simulink library "senseo_lib"  (R2018a)
settings: Solver=VariableStepAuto  StartTime=0.0  StopTime=10.0  RelTol=1e-3
libraries: fl_lib x10, elec_lib x8, $bdroot x2
settings Model: Creator=ChLan  LastModifiedBy=ChLan

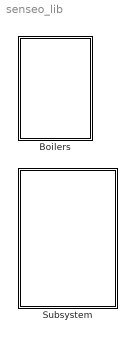
== system senseo_lib ==
  Boilers : Subsystem
  Subsystem : Subsystem

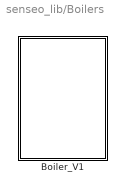
== system senseo_lib/Boilers ==
  Boiler_V1 : Subsystem

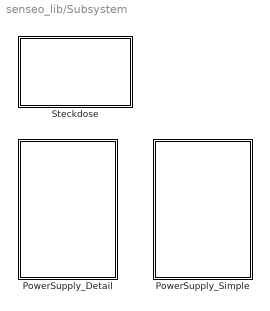
== system senseo_lib/Subsystem ==
  PowerSupply_Detail : Subsystem
  PowerSupply_Simple : Subsystem  VariantControl=1==1
  Steckdose : Subsystem

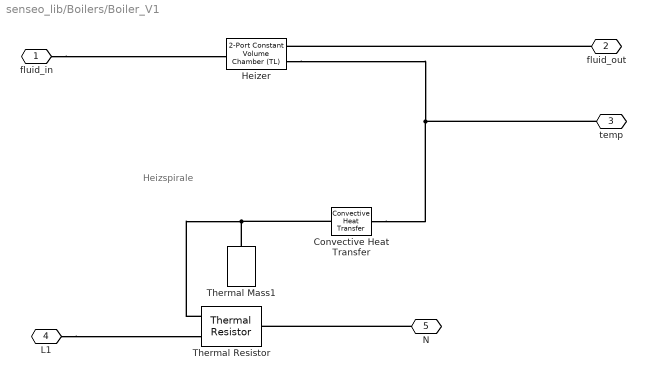
== system senseo_lib/Boilers/Boiler_V1 ==
  note: Heizspirale
  Convective Heat Transfer : fl_lib/Thermal/Thermal Elements/Convective Heat Transfer  area=1000 cm^2  heat_tr_coeff=1000 W/(m^2 * K)  T_specify=off  T_priority=None  T=0 K  T_nominal_specify=off  T_nominal_unit=K  T_nominal_value=1  Q_specify=off  Q_priority=None  Q=0 W  Q_nominal_specify=off  Q_nominal_unit=W  Q_nominal_value=1
  Heizer : fl_lib/Thermal Liquid/Elements/2-Port Constant Volume Chamber (TL)  volume=0.25 l  area_A=0.01 m^2  area_B=0.01 m^2  p_chamber_specify=off  p_chamber_priority=High  p_chamber=0.101325 MPa  p_chamber_nominal_specify=off  p_chamber_nominal_unit=MPa  p_chamber_nominal_value=1  T_chamber_specify=on  T_chamber_priority=High  T_chamber=300 K  T_chamber_nominal_specify=off  T_chamber_nominal_unit=K  T_chamber_nominal_value=1  u_chamber_specify=off  u_chamber_priority=None  u_chamber=83.90600000000001 kJ/kg  u_chamber_nominal_specify=off  u_chamber_nominal_unit=kJ/kg  u_chamber_nominal_value=1  rho_specify=off  rho_priority=None  rho=998.21 kg/m^3  rho_nominal_specify=off  rho_nominal_unit=kg/m^3  rho_nominal_value=1
      settings: SourceProductName=Simscape  SourceProductBaseCode=SS
  Thermal Mass1 : fl_lib/Thermal/Thermal Elements/Thermal Mass  mass=0.05 kg  sp_heat=447 J/kg/K  T_specify=off  T_priority=High  T=300 K  T_nominal_specify=off  T_nominal_unit=K  T_nominal_value=1  Q_specify=off  Q_priority=None  Q=0 W  Q_nominal_specify=off  Q_nominal_unit=W  Q_nominal_value=1
  Thermal Resistor : fl_lib/Electrical/Electrical Elements/Thermal Resistor  R0=35 Ohm  T0=298.15 K  alpha=50e-6 1/K  tc=10 s  K_d=1e-3 W/K  T_specify=off  T_priority=High  T=300 K  T_nominal_specify=off  T_nominal_unit=K  T_nominal_value=1
      settings: SourceProductName=Simscape  SourceProductBaseCode=SS
  fluid_in : PMIOPort  Side=Left
  fluid_out : PMIOPort  Port=2  Side=Right
  temp : PMIOPort  Port=3  Side=Right
  L1 : PMIOPort  Port=4  Side=Left
  N : PMIOPort  Port=5  Side=Right
  connections:
  fluid_in/RConn1 -- Heizer/RConn1
  fluid_out/RConn1 -- Heizer/LConn1
  N/RConn1 -- Thermal Resistor/RConn1
  Convective Heat Transfer/LConn1 -- Thermal Mass1/LConn1 -- Thermal Resistor/LConn1
  temp/RConn1 -- Heizer/LConn2 -- Convective Heat Transfer/RConn1
  L1/RConn1 -- Thermal Resistor/LConn2

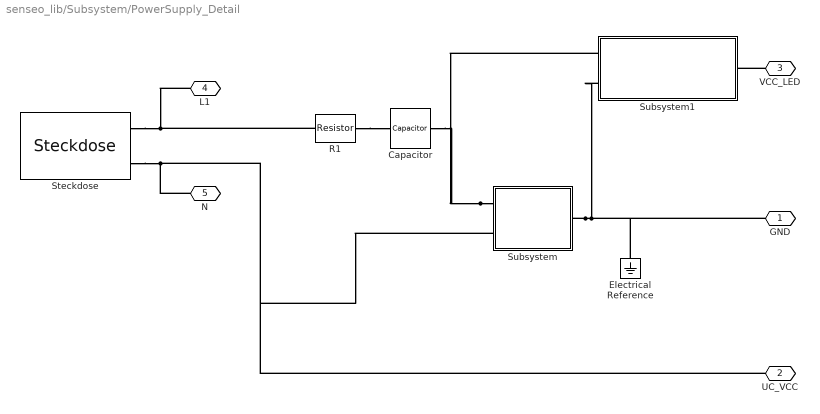
== system senseo_lib/Subsystem/PowerSupply_Detail ==
  Capacitor : elec_lib/Passive Devices/Capacitor  enable_table=0  c=680 nF  Cvec=[1e-05, 1e-06] F  Vvec=[0, 10] V  CV_table_symmetry=1  C_tol=5  enable_C_tol=0  tol_distribution=1  nSigma=4  r=1e-6 Ohm  g=0 1/Ohm  enable_operating_limits=0  operating_limit_action=2  max_working_voltage_range=[-25, 25] V  power_rating=1 W  enable_faults=0  fault_action=1  Cscale_faulted=100  R_faulted=1e-3 Ohm  G_faulted=0 1/Ohm  tau_fault=1e-3 s  enable_temporal_fault=0  t_fault=1 s  enable_behavioral_fault=0  max_permissible_voltage_range=[-100, 100] V  t_fail_on_voltage=1 s  i_specify=off  i_priority=None  i=0 A  i_nominal_specify=off  i_nominal_unit=A  i_nominal_value=1  v_specify=off  v_priority=None  v=0 V  v_nominal_specify=off  v_nominal_unit=V  v_nominal_value=1  vc_specify=off  vc_priority=High  vc=0 V  vc_nominal_specify=off  vc_nominal_unit=V  vc_nominal_value=1
      settings: AttributesFormatString=%<c> %<c_unit>
  Electrical Reference : fl_lib/Electrical/Electrical Elements/Electrical Reference
  R1 : elec_lib/Passive Devices/Resistor  R=100 Ohm  R_tol=5  enable_R_tol=0  tol_distribution=1  nSigma=4  enable_operating_limits=0  operating_limit_action=2  max_working_voltage=100 V  power_rating=1 W  enable_faults=0  fault_action=1  R_faulted=inf Ohm  enable_temporal_fault=0  t_fault=1 s  enable_behavioral_fault=0  max_permissible_current=1 A  t_fail_on_current=1 s  noise_mode=0  sample_time=1e-3 s  repeatability=1  auto_seed=1399327243  user_seed=0  Tdevice=25 degC  alpha=3.93e-3 1/K  Tmeas=25 degC  thermal_mass=100 J/K  power_derating_T1=70 degC  power_derating_T2=155 degC  operating_temperature_range_vec=[-50, 150] degC  temperature_specify=off  temperature_priority=High  temperature=298.15 K  temperature_nominal_specify=off  temperature_nominal_unit=K  temperature_nominal_value=1
      settings: AttributesFormatString="%<R>  %<R_unit>"
  Steckdose : $bdroot/Subsystem/Steckdose
  Subsystem : Subsystem
  Subsystem1 : Subsystem
  GND : PMIOPort  Side=Right
  UC_VCC : PMIOPort  Port=2  Side=Right
  VCC_LED : PMIOPort  Port=3  Side=Right
  L1 : PMIOPort  Port=4  Side=Right
  N : PMIOPort  Port=5  Side=Right
  connections:
  R1/LConn1 -- Steckdose/RConn1 -- L1/RConn1
  R1/RConn1 -- Capacitor/LConn1
  UC_VCC/RConn1 -- Subsystem/LConn2 -- Steckdose/RConn2 -- N/RConn1
  Subsystem/RConn1 -- Electrical Reference/LConn1 -- GND/RConn1 -- Subsystem1/LConn2
  Subsystem/LConn1 -- Capacitor/RConn1 -- Subsystem1/LConn1
  VCC_LED/RConn1 -- Subsystem1/RConn1

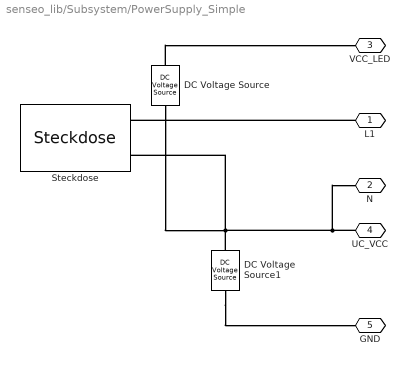
== system senseo_lib/Subsystem/PowerSupply_Simple ==
  DC Voltage Source : fl_lib/Electrical/Electrical Sources/DC Voltage Source  v0=12 V
  DC Voltage Source1 : fl_lib/Electrical/Electrical Sources/DC Voltage Source  v0=5.1 V
  Steckdose : $bdroot/Subsystem/Steckdose
  L1 : PMIOPort  Side=Right
  N : PMIOPort  Port=2  Side=Right
  VCC_LED : PMIOPort  Port=3  Side=Right
  UC_VCC : PMIOPort  Port=4  Side=Right
  GND : PMIOPort  Port=5  Side=Right
  connections:
  DC Voltage Source/LConn1 -- VCC_LED/RConn1
  DC Voltage Source1/LConn1 -- Steckdose/RConn2 -- DC Voltage Source/RConn1 -- UC_VCC/RConn1 -- N/RConn1
  DC Voltage Source1/RConn1 -- GND/RConn1
  L1/RConn1 -- Steckdose/RConn1

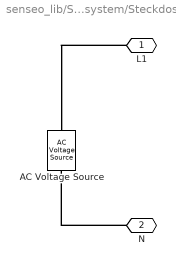
== system senseo_lib/Subsystem/Steckdose ==
  AC Voltage Source : fl_lib/Electrical/Electrical Sources/AC Voltage Source  amp=230 * sqrt(2) V  shift=0 deg  frequency=50 Hz  omega=0 rad/s
      settings: AttributesFormatString=|
      | %<amp> %<amp_unit>
      | %<frequency> %<frequency_unit>
  L1 : PMIOPort  Side=Right
  N : PMIOPort  Port=2  Side=Right
  connections:
  N/RConn1 -- AC Voltage Source/RConn1
  L1/RConn1 -- AC Voltage Source/LConn1

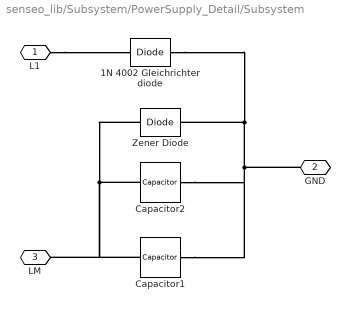
== system senseo_lib/Subsystem/PowerSupply_Detail/Subsystem ==
  1N 4002 Gleichrichterdiode : fl_lib/Electrical/Electrical Elements/Diode  Vf=0.6 V  Ron=0.3 Ohm  Goff=1e-8 1/Ohm  i_specify=off  i_priority=None  i=0 A  i_nominal_specify=off  i_nominal_unit=A  i_nominal_value=1  v_specify=off  v_priority=None  v=0 V  v_nominal_specify=off  v_nominal_unit=V  v_nominal_value=1
  Capacitor1 : elec_lib/Passive Devices/Capacitor  enable_table=0  c=470 uF  Cvec=[1e-05, 1e-06] F  Vvec=[0, 10] V  CV_table_symmetry=1  C_tol=5  enable_C_tol=0  tol_distribution=1  nSigma=4  r=1e-6 Ohm  g=0 1/Ohm  enable_operating_limits=0  operating_limit_action=2  max_working_voltage_range=[-25, 25] V  power_rating=1 W  enable_faults=0  fault_action=1  Cscale_faulted=100  R_faulted=1e-3 Ohm  G_faulted=0 1/Ohm  tau_fault=1e-3 s  enable_temporal_fault=0  t_fault=1 s  enable_behavioral_fault=0  max_permissible_voltage_range=[-100, 100] V  t_fail_on_voltage=1 s  i_specify=off  i_priority=None  i=0 A  i_nominal_specify=off  i_nominal_unit=A  i_nominal_value=1  v_specify=off  v_priority=None  v=0 V  v_nominal_specify=off  v_nominal_unit=V  v_nominal_value=1  vc_specify=off  vc_priority=High  vc=0 V  vc_nominal_specify=off  vc_nominal_unit=V  vc_nominal_value=1
      settings: AttributesFormatString=%<c> %<c_unit>
  Capacitor2 : elec_lib/Passive Devices/Capacitor  enable_table=0  c=100 nF  Cvec=[1e-05, 1e-06] F  Vvec=[0, 10] V  CV_table_symmetry=1  C_tol=5  enable_C_tol=0  tol_distribution=1  nSigma=4  r=1e-6 Ohm  g=0 1/Ohm  enable_operating_limits=0  operating_limit_action=2  max_working_voltage_range=[-25, 25] V  power_rating=1 W  enable_faults=0  fault_action=1  Cscale_faulted=100  R_faulted=1e-3 Ohm  G_faulted=0 1/Ohm  tau_fault=1e-3 s  enable_temporal_fault=0  t_fault=1 s  enable_behavioral_fault=0  max_permissible_voltage_range=[-100, 100] V  t_fail_on_voltage=1 s  i_specify=off  i_priority=None  i=0 A  i_nominal_specify=off  i_nominal_unit=A  i_nominal_value=1  v_specify=off  v_priority=None  v=0 V  v_nominal_specify=off  v_nominal_unit=V  v_nominal_value=1  vc_specify=off  vc_priority=High  vc=0 V  vc_nominal_specify=off  vc_nominal_unit=V  vc_nominal_value=1
      settings: AttributesFormatString=%<c> %<c_unit>
  Zener Diode : elec_lib/Semiconductor Devices/Diode  ModelType=2  Vf=5.1 V  Ron=0.3 Ohm  Goff=1e-8 S  Rz=0.3 Ohm  Vz=50 V  C_PWL=5 pF  prmExp=1  I12=[.0137, .545] A  V12=[.6, .7] V  I1=0.0137 A  V1=0.6 V  IS=1e-12 A  ec=1  RS=0.01 Ohm  Tmeas=25 degC  BV=inf V  C_param=1  CJ0=5 pF  VJ=1 V  Mgrad=0.5  Vvec=[.1, 10, 100] V  Cvec=[3.5, 1, .4] pF  FC=0.5  Q_param=1  Irrm=-7.15 A  iF=4 A  didt=-750 A/us  trr=115 ns  TT=50 ns  tau=100 ns  T_param=1  IS_T2=1.25e-7 A  I1_T2=0.245 A  V1_T2=0.5 V  Tmeas2=125 degC  EG_param=1  EG=1.11 eV  XTI_param=1  XTI=3  dBVdT=0 V/K  Tdevice=25 degC  i_capacitor_specify=off  i_capacitor_priority=High  i_capacitor=0 A  i_capacitor_nominal_specify=off  i_capacitor_nominal_unit=A  i_capacitor_nominal_value=1  v_capacitor_specify=off  v_capacitor_priority=None  v_capacitor=0 V  v_capacitor_nominal_specify=off  v_capacitor_nominal_unit=V  v_capacitor_nominal_value=1  Rth=[0, 10] K/W  thermal_mass_parameterization=1  thermal_mass=[0, 1] J/K  thermal_time_constant=[0, 10] s  thermal_mass_initial_temperatures=[25, 25] degC
      settings: SourceProductName=Simscape Electronics  SourceProductBaseCode=SN
  L1 : PMIOPort  Side=Left
  GND : PMIOPort  Port=2  Side=Right
  LM : PMIOPort  Port=3  Side=Left
  connections:
  Zener Diode/RConn1 -- Capacitor2/LConn1 -- Capacitor1/LConn1 -- LM/RConn1
  1N 4002 Gleichrichterdiode/LConn1 -- Zener Diode/LConn1 -- Capacitor2/RConn1 -- Capacitor1/RConn1 -- GND/RConn1
  L1/RConn1 -- 1N 4002 Gleichrichterdiode/RConn1

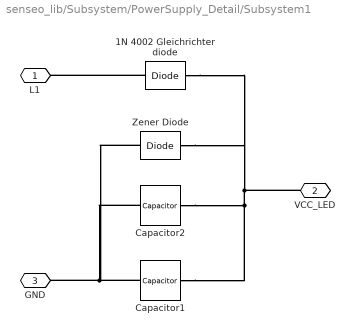
== system senseo_lib/Subsystem/PowerSupply_Detail/Subsystem1 ==
  1N 4002 Gleichrichterdiode : fl_lib/Electrical/Electrical Elements/Diode  Vf=0.6 V  Ron=0.3 Ohm  Goff=1e-8 1/Ohm  i_specify=off  i_priority=None  i=0 A  i_nominal_specify=off  i_nominal_unit=A  i_nominal_value=1  v_specify=off  v_priority=None  v=0 V  v_nominal_specify=off  v_nominal_unit=V  v_nominal_value=1
  Capacitor1 : elec_lib/Passive Devices/Capacitor  enable_table=0  c=470 uF  Cvec=[1e-05, 1e-06] F  Vvec=[0, 10] V  CV_table_symmetry=1  C_tol=5  enable_C_tol=0  tol_distribution=1  nSigma=4  r=1e-6 Ohm  g=0 1/Ohm  enable_operating_limits=0  operating_limit_action=2  max_working_voltage_range=[-25, 25] V  power_rating=1 W  enable_faults=0  fault_action=1  Cscale_faulted=100  R_faulted=1e-3 Ohm  G_faulted=0 1/Ohm  tau_fault=1e-3 s  enable_temporal_fault=0  t_fault=1 s  enable_behavioral_fault=0  max_permissible_voltage_range=[-100, 100] V  t_fail_on_voltage=1 s  i_specify=off  i_priority=None  i=0 A  i_nominal_specify=off  i_nominal_unit=A  i_nominal_value=1  v_specify=off  v_priority=None  v=0 V  v_nominal_specify=off  v_nominal_unit=V  v_nominal_value=1  vc_specify=off  vc_priority=High  vc=0 V  vc_nominal_specify=off  vc_nominal_unit=V  vc_nominal_value=1
      settings: AttributesFormatString=%<c> %<c_unit>
  Capacitor2 : elec_lib/Passive Devices/Capacitor  enable_table=0  c=100 nF  Cvec=[1e-05, 1e-06] F  Vvec=[0, 10] V  CV_table_symmetry=1  C_tol=5  enable_C_tol=0  tol_distribution=1  nSigma=4  r=1e-6 Ohm  g=0 1/Ohm  enable_operating_limits=0  operating_limit_action=2  max_working_voltage_range=[-25, 25] V  power_rating=1 W  enable_faults=0  fault_action=1  Cscale_faulted=100  R_faulted=1e-3 Ohm  G_faulted=0 1/Ohm  tau_fault=1e-3 s  enable_temporal_fault=0  t_fault=1 s  enable_behavioral_fault=0  max_permissible_voltage_range=[-100, 100] V  t_fail_on_voltage=1 s  i_specify=off  i_priority=None  i=0 A  i_nominal_specify=off  i_nominal_unit=A  i_nominal_value=1  v_specify=off  v_priority=None  v=0 V  v_nominal_specify=off  v_nominal_unit=V  v_nominal_value=1  vc_specify=off  vc_priority=High  vc=0 V  vc_nominal_specify=off  vc_nominal_unit=V  vc_nominal_value=1
      settings: AttributesFormatString=%<c> %<c_unit>
  Zener Diode : elec_lib/Semiconductor Devices/Diode  ModelType=2  Vf=5.1 V  Ron=0.3 Ohm  Goff=1e-8 S  Rz=0.3 Ohm  Vz=50 V  C_PWL=5 pF  prmExp=1  I12=[.0137, .545] A  V12=[.6, .7] V  I1=0.0137 A  V1=0.6 V  IS=1e-12 A  ec=1  RS=0.01 Ohm  Tmeas=25 degC  BV=inf V  C_param=1  CJ0=5 pF  VJ=1 V  Mgrad=0.5  Vvec=[.1, 10, 100] V  Cvec=[3.5, 1, .4] pF  FC=0.5  Q_param=1  Irrm=-7.15 A  iF=4 A  didt=-750 A/us  trr=115 ns  TT=50 ns  tau=100 ns  T_param=1  IS_T2=1.25e-7 A  I1_T2=0.245 A  V1_T2=0.5 V  Tmeas2=125 degC  EG_param=1  EG=1.11 eV  XTI_param=1  XTI=3  dBVdT=0 V/K  Tdevice=25 degC  i_capacitor_specify=off  i_capacitor_priority=High  i_capacitor=0 A  i_capacitor_nominal_specify=off  i_capacitor_nominal_unit=A  i_capacitor_nominal_value=1  v_capacitor_specify=off  v_capacitor_priority=None  v_capacitor=0 V  v_capacitor_nominal_specify=off  v_capacitor_nominal_unit=V  v_capacitor_nominal_value=1  Rth=[0, 10] K/W  thermal_mass_parameterization=1  thermal_mass=[0, 1] J/K  thermal_time_constant=[0, 10] s  thermal_mass_initial_temperatures=[25, 25] degC
      settings: SourceProductName=Simscape Electronics  SourceProductBaseCode=SN
  L1 : PMIOPort  Side=Left
  VCC_LED : PMIOPort  Port=2  Side=Right
  GND : PMIOPort  Port=3  Side=Left
  connections:
  Capacitor1/LConn1 -- GND/RConn1 -- Capacitor2/LConn1 -- Zener Diode/LConn1
  Capacitor2/RConn1 -- Capacitor1/RConn1 -- VCC_LED/RConn1 -- 1N 4002 Gleichrichterdiode/RConn1 -- Zener Diode/RConn1
  1N 4002 Gleichrichterdiode/LConn1 -- L1/RConn1
